simulink model "BoostConverterTestEnviroment"  (R2020a)
settings: Solver=ode15s  StartTime=0.0  StopTime=0.05  RelTol=1e-3
libraries: ee_lib x2, fl_lib x1, nesl_utility x1
settings Model: Creator=ykamatan  LastModifiedBy=ykamatan
settings SolverCC: MaxConsecutiveMinStep=10
settings DataIOCC: SaveOutput=off  SaveTime=off

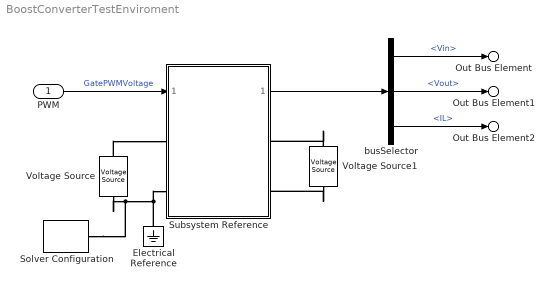
== system BoostConverterTestEnviroment ==
  PWM : Inport  OutDataTypeStr=double  PortDimensions=1  SampleTime=[2e-08,0]
  Electrical Reference : fl_lib/Electrical/Electrical Elements/Electrical Reference
  Solver Configuration : nesl_utility/Solver Configuration  PhysicalDomain=network_engine_domain  SubClassName=solver  LeftPortType=input  RightPortType=generic  Tones=[]  Harmonics=[]  SimulateNoise=off  Profile=off  UseLocalSampling=off  EnableSwitchedLinearOptims=on  FrequencyDomain=off  UseCCode=off  RelTol=0.001  AbsTol=1e-06  MinStep=1e-09  ToWorkspace=off  RevertToSquareIcSolve=off  NumHomotopyIterations=100  PhasorMode=off  PhasorModeNumHarmonics=1  DoDC=off  ResidualTolerance=1e-09  UseLocalSolver=off  LocalSolverChoice=NE_BACKWARD_EULER_ADVANCER  LocalSolverSampleTime=0.001  DoFixedCost=off  MaxNonlinIter=3  MaxModeIter=2  LinearAlgebra=auto  EquationFormulation=NE_TIME_EF  DelaysMemoryBudget=1024  AutomaticFiltering=on  FilteringTimeConstant=0.001  PartitionStorageMethod=AS_NEEDED  PartitionMemoryBudget=1024  PartitionMethod=ROBUST
  Subsystem Reference : Subsystem  ReferencedSubsystem=BoostConverter
  Voltage Source : ee_lib/Sources/Voltage Source  dc_voltage=100 V  ac_voltage=0 V  ac_shift=0 rad  ac_frequency=60 Hz  noise_mode=0  PSD=0 V^2/Hz  repeatability=1  auto_seed=1811450916  user_seed=0  sample_time=1e-3 s  i_specify=off  i_priority=None  i=0 A  i_nominal_specify=off  i_nominal_unit=A  i_nominal_value=1  v_specify=off  v_priority=None  v=0 V  v_nominal_specify=off  v_nominal_unit=V  v_nominal_value=1
  Voltage Source1 : ee_lib/Sources/Voltage Source  dc_voltage=320 V  ac_voltage=0 V  ac_shift=0 rad  ac_frequency=60 Hz  noise_mode=0  PSD=0 V^2/Hz  repeatability=1  auto_seed=3933054132  user_seed=0  sample_time=1e-3 s  i_specify=off  i_priority=None  i=0 A  i_nominal_specify=off  i_nominal_unit=A  i_nominal_value=1  v_specify=off  v_priority=None  v=0 V  v_nominal_specify=off  v_nominal_unit=V  v_nominal_value=1
  busSelector : BusSelector  OutputSignals=Vin,Vout,IL
  Out Bus Element : Outport  PortName=Signals  Element=Vin
  Out Bus Element1 : Outport  PortName=Signals  Element=Vout
  Out Bus Element2 : Outport  PortName=Signals  Element=IL
  wires:
  busSelector/3 -> Out Bus Element2/1  "<IL>"
  busSelector/2 -> Out Bus Element1/1  "<Vout>"
  busSelector/1 -> Out Bus Element/1  "<Vin>"
  Subsystem Reference/1 -> busSelector/1
  PWM/1 -> Subsystem Reference/1  "GatePWMVoltage"
  connections:
  Voltage Source/RConn1 -- Subsystem Reference/LConn2 -- Electrical Reference/LConn1 -- Solver Configuration/RConn1
  Voltage Source1/RConn1 -- Subsystem Reference/RConn2
  Voltage Source/LConn1 -- Subsystem Reference/LConn1
  Voltage Source1/LConn1 -- Subsystem Reference/RConn1
